simulink model "AHM_loop"  (R2024a)
settings: Solver=FixedStepDiscrete  StartTime=0.0  StopTime=TMax  FixedStep=dt  RelTol=1e-3
PreLoadFcn:
  | initializeSimulation
  | initializeSCRAMNetGT
settings Model: Creator=mvetsch  LastModifiedBy=mcdevin
settings SolverCC: AlgebraicLoopSolver=TrustRegion
settings DataIOCC: SaveFormat=Array  SaveOutput=off  SignalLogging=off  SaveTime=off  ReturnWorkspaceOutputs=off  SignalLoggingName=sigsOut
settings OptimizationCC: BlockReduction=off  OptimizeBlockIOStorage=off  BufferReuse=off  GlobalBufferReuse=off  ExpressionFolding=off  ExpressionDepthLimit=2147483647  LocalBlockOutputs=off  InitFltsAndDblsToZero=on  EfficientFloat2IntCast=on  LifeSpan=inf  SimCompilerOptimization=on  OptimizeDataStoreBuffers=off  BusAssignmentInplaceUpdate=off
settings DebuggingCC: SaveWithParameterizedLinksMsg=none  CheckSSInitialOutputMsg=off  UnderspecifiedInitializationDetection=Classic  MergeDetectMultiDrivingBlocksExec=none  UnconnectedInputMsg=warning  UnconnectedOutputMsg=warning  UnconnectedLineMsg=warning  AllowSymbolicDim=off  StateNameClashWarn=warning  PregeneratedLibrarySubsystemCodeDiagnostic=none  SFUnexpectedBacktrackingDiag=warning  SFNoUnconditionalDefaultTransitionDiag=warning  SFExecutionAtInitializationDiag=none  ArithmeticOperatorsInVariantConditions=warning
settings HardwareCC: ProdBitPerPointer=32  ProdBitPerSizeT=32  ProdBitPerPtrDiffT=32  ProdLargestAtomicFloat=None  ProdWordSize=32  ProdLongLongMode=on  ProdHWDeviceType=Generic->32-bit x86 compatible  TargetHWDeviceType=32-bit Generic
settings ModelReferenceCC: EnableRefExpFcnMdlSchedulingChecks=on  PropagateSignalLabelsOutOfModel=off
settings SFSimCC: SimCustomHeaderCode="#include \"PredictorCorrector.h\""  SimUserSources=PredictorCorrector.c  SimUserIncludeDirs="\"C:\\Program Files\\OpenFresco\\SourceCode\\SRC\\experimentalControl\\Simulink\\HybridSimToolbox\""  SimUseLocalCustomCode=off  SimParseCustomCode=off  CustomCodeUndefinedFunction=UseInterfaceOnly
settings RTWCC: Description=Simulink Real-Time  SystemTargetFile=slrt.tlc  TemplateMakefile=slrt_default_tmf  RTWUseLocalCustomCode=off  CustomHeaderCode="#include \"PredictorCorrector.h\""  CustomSource=PredictorCorrector.c  RTWCompilerOptimization=on  GPUComputeCapability=3.5
settings RTWCC: CustomInclude=|
  | "C:\Program Files\OpenFresco\SourceCode\SRC\experimentalControl\Simulink\HybridSimToolbox"
  | "C:\Projects\Michael\openfast\build\bin"
settings CodeAppCC: StateflowObjectComments=on
settings SimulinkRealTimeCC: TargetFcnLib=ansi_tfl_tmw.mat  InstructionSetFMA=off  OptimizeReductions=off  LogToMDFFile=off
settings ConfigComp: CovMetricSettings=dw  CovSaveCumulativeToWorkspaceVar=on  CovSaveSingleToWorkspaceVar=on  CovExternalEMLEnable=off

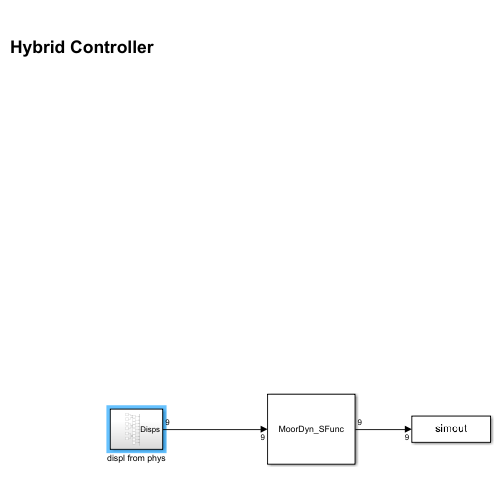
[thumbnail: Simulink's stored preview of the top-level diagram]
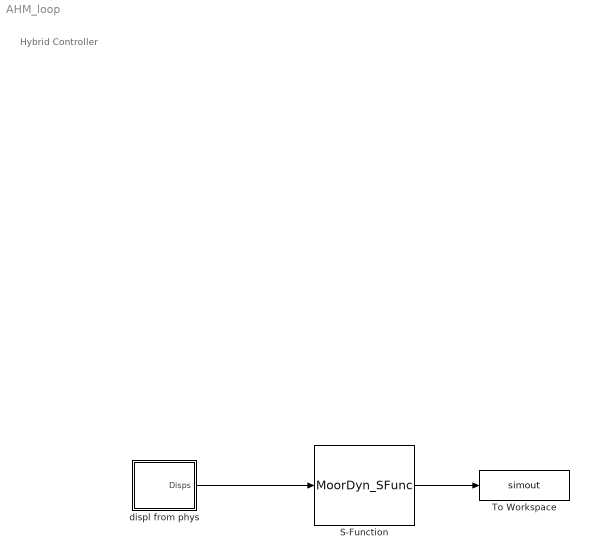
== system AHM_loop ==
  note: Hybrid Controller
  S-Function : S-Function  FunctionName=MoorDyn_SFunc  Parameters=MD_InputFileName, dt, TMax  SFunctionDeploymentMode=off  EnableBusSupport=off
  To Workspace : ToWorkspace  VariableName=simout  SaveFormat=Timeseries  SampleTime=-1
  displ from phys : Subsystem
  wires:
  displ from phys/1(Disps) -> S-Function/1
  S-Function/1 -> To Workspace/1

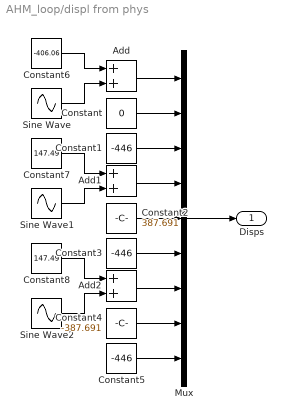
== system AHM_loop/displ from phys ==
  Add : Sum
  Add1 : Sum
  Add2 : Sum
  Constant : Constant  Value=0
  Constant1 : Constant  Value=-446
  Constant2 : Constant  Value=387.691
  Constant3 : Constant  Value=-446
  Constant4 : Constant  Value=-387.691
  Constant5 : Constant  Value=-446
  Constant6 : Constant  Value=-406.06
  Constant7 : Constant  Value=147.49
  Constant8 : Constant  Value=147.49
  Mux : Mux  Inputs=9
  Sine Wave : Sin  Amplitude=5  Frequency=0.314159265358979323846  SampleTime=0
  Sine Wave1 : Sin  Amplitude=5  Frequency=0.314159265358979323846  SampleTime=0
  Sine Wave2 : Sin  Amplitude=5  Frequency=0.314159265358979323846  SampleTime=0
  Disps : Outport  VectorParamsAs1DForOutWhenUnconnected=off
  wires:
  Constant3/1 -> Mux/6
  Constant2/1 -> Mux/5
  Constant/1 -> Mux/2
  Constant1/1 -> Mux/3
  Mux/1 -> Disps/1
  Constant4/1 -> Mux/8
  Constant5/1 -> Mux/9
  Add/1 -> Mux/1
  Add1/1 -> Mux/4
  Add2/1 -> Mux/7
  Sine Wave/1 -> Add/2
  Constant6/1 -> Add/1
  Constant7/1 -> Add1/1
  Sine Wave1/1 -> Add1/2
  Constant8/1 -> Add2/1
  Sine Wave2/1 -> Add2/2
